simulink model "PTOEnblSwt_DD"  (R2016b)
settings: configuration reference "CodeGenConfigSet" (kept outside this file)
values from neighbouring files (symbols this model uses):
  PTOEnblSwt_stDflVal_C = Calibration.Parameter    [init_PTOEnblSwt_DD.m]    (also in init_PTOEnblSwt_DD_SIL.m = Simulink.Parameter)
  PTOEnblSwt_swtSigSel_C = Calibration.Parameter    [init_PTOEnblSwt_DD.m]    (also in init_PTOEnblSwt_DD_SIL.m = Simulink.Parameter)
  PTOEnblSwt_tiDebHiLo_C = Calibration.Parameter    [init_PTOEnblSwt_DD.m]    (also in init_PTOEnblSwt_DD_SIL.m = Simulink.Parameter)
  PTOEnblSwt_tiDebLoHi_C = Calibration.Parameter    [init_PTOEnblSwt_DD.m]    (also in init_PTOEnblSwt_DD_SIL.m = Simulink.Parameter)
undefined symbols (not defined in the file or in its folder): PTOEnblSwt_DD_DT, Switch_conv
libraries: CXLib x1
settings Model: Creator=bianxuyin  LastModifiedBy=bianxuyin
settings ConfigSetRef: SourceLocation=Base Workspace

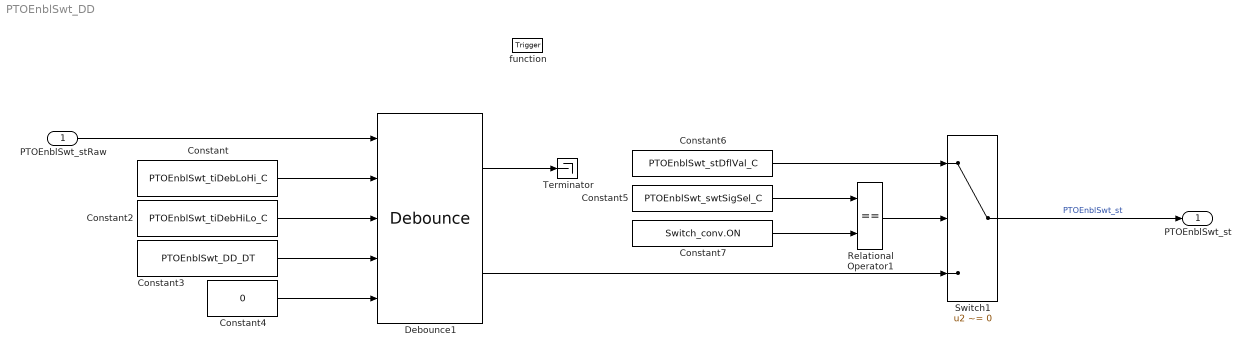
== system PTOEnblSwt_DD ==
  PTOEnblSwt_stRaw : Inport  Description=PTO enable switch Raw  OutMin=0  OutMax=1  OutDataTypeStr=boolean
  function : TriggerPort  TriggerType=function-call  VariantControl=Variant
  Constant : Constant  Value=PTOEnblSwt_tiDebLoHi_C
  Constant2 : Constant  Value=PTOEnblSwt_tiDebHiLo_C
  Constant3 : Constant  Value=PTOEnblSwt_DD_DT
  Constant4 : Constant  Value=0  OutDataTypeStr=Inherit: Inherit via back propagation
  Constant5 : Constant  Value=PTOEnblSwt_swtSigSel_C
  Constant6 : Constant  Value=PTOEnblSwt_stDflVal_C
  Constant7 : Constant  Value=Switch_conv.ON
  Debounce1 : CXLib/Debounce
  Relational Operator1 : RelationalOperator  Operator===  OutDataTypeStr=boolean  RndMeth=Nearest
  Switch1 : Switch  Criteria=u2 ~= 0  InputSameDT=on
  Terminator : Terminator
  PTOEnblSwt_st : Outport  Description=PTO enable switch status  OutMin=0  OutMax=1  OutDataTypeStr=boolean
  wires:
  Switch1/1 -> PTOEnblSwt_st/1  "PTOEnblSwt_st"
  Constant6/1 -> Switch1/1
  Debounce1/1 -> Terminator/1
  Constant2/1 -> Debounce1/3
  Constant4/1 -> Debounce1/5
  Constant/1 -> Debounce1/2
  PTOEnblSwt_stRaw/1 -> Debounce1/1
  Constant7/1 -> Relational Operator1/2
  Relational Operator1/1 -> Switch1/2
  Constant5/1 -> Relational Operator1/1
  Debounce1/2 -> Switch1/3
  Constant3/1 -> Debounce1/4
